simulink model "PS10_template2023"  (R2022b)
settings: Solver=ode45  StartTime=0.0  StopTime=10  FixedStep=.002  RelTol=1e-3  EnableMultiTasking=on
settings Model: ExtModeTrigDuration=10000  Creator=smascaro  LastModifiedBy=willg
settings SolverCC: AlgebraicLoopSolver=TrustRegion  PositivePriorityOrder=on
settings DataIOCC: SaveFormat=Array  SignalLoggingSaveFormat=ModelDataLogs  SaveOutput=off  SaveTime=off  ReturnWorkspaceOutputs=off
settings OptimizationCC: ExpressionDepthLimit=2147483647  InitFltsAndDblsToZero=on  LifeSpan=inf
settings DebuggingCC: SaveWithParameterizedLinksMsg=none  UnderspecifiedInitializationDetection=Classic  MergeDetectMultiDrivingBlocksExec=none  SignalResolutionControl=TryResolveAllWithWarning  SolverPrmCheckMsg=warning  MultiTaskDSMMsg=warning  MultiTaskCondExecSysMsg=none  FcnCallInpInsideContextMsg=warning  UnconnectedInputMsg=warning  UnconnectedOutputMsg=warning  UnconnectedLineMsg=warning  AllowSymbolicDim=off  StateNameClashWarn=warning  SFUnexpectedBacktrackingDiag=warning  SFNoUnconditionalDefaultTransitionDiag=warning  SFExecutionAtInitializationDiag=none  SFMachineParentedDataDiag=warning  ArithmeticOperatorsInVariantConditions=warning
settings HardwareCC: ProdBitPerPointer=32  ProdBitPerSizeT=32  ProdBitPerPtrDiffT=32  ProdLargestAtomicFloat=None  ProdIntDivRoundTo=Undefined  ProdEndianess=Unspecified  ProdWordSize=32  ProdHWDeviceType=32-bit Generic  TargetBitPerPointer=64  TargetBitPerSizeT=64  TargetBitPerPtrDiffT=64  TargetLongLongMode=on  TargetIntDivRoundTo=Zero  TargetEndianess=LittleEndian  TargetWordSize=64  TargetHWDeviceType=MATLAB Host
settings ModelReferenceCC: EnableRefExpFcnMdlSchedulingChecks=on  PropagateSignalLabelsOutOfModel=off
settings SFSimCC: SimUseLocalCustomCode=off  SimParseCustomCode=off  CustomCodeUndefinedFunction=UseInterfaceOnly
settings RTWCC: Description=QUARC Win32 Target  SystemTargetFile=quarc_windows.tlc  TemplateMakefile=quarc_default_tmf  RTWUseLocalCustomCode=off  DLArmComputeVersion=19.05
settings CodeAppCC: StateflowObjectComments=on
settings STFCustomTargetCC: TargetPreCompLibLocation=C:\PROGRA~3\QUARC\lib\2018a\windows\release  CPPClassGenCompliant=on  GRTInterface=on  SystemTargetFile=quarc_windows.tlc
settings GRTTargetCC: TargetPreCompLibLocation=C:\PROGRA~3\QUARC\lib\2018a\windows\release  TargetLangStandard=C89/C90 (ANSI)  ParMdlRefBuildCompliant=off  CompOptLevelCompliant=off  ConcurrentExecutionCompliant=off  CombineOutputUpdateFcns=off  MatFileLogging=off  GRTInterface=on  UseToolchainInfoCompliant=off  ExtMode=on  ExtModeMexFile=quarc_comm
settings ConfigComp: CovMetricSettings=dw  CovSaveCumulativeToWorkspaceVar=on  CovSaveSingleToWorkspaceVar=on  CovExternalEMLEnable=off

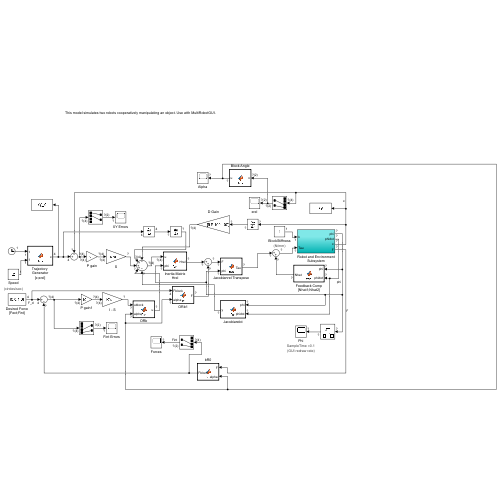
[thumbnail: Simulink's stored preview of the top-level diagram]
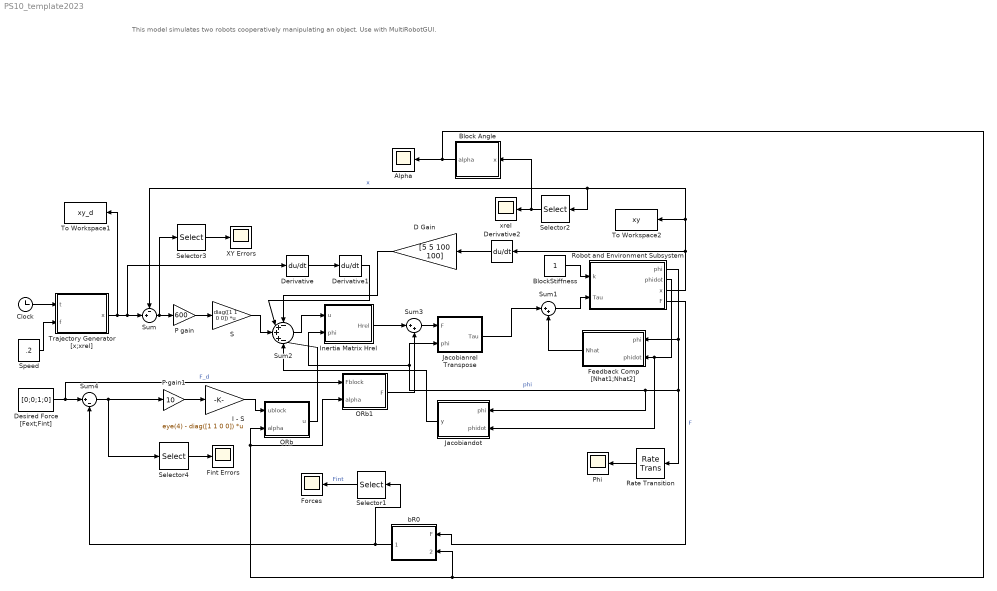
== system PS10_template2023 ==
  note: This model simulates two robots cooperatively manipulating an object. Use with MultiRobotGUI.
  Alpha : Scope
  Block Angle : MATLAB Function  TreatAsAtomicUnit=on
  BlockStiffness : Constant
      settings: AttributesFormatString=(N/mm)
  Clock : Clock
  D Gain : Gain  Gain=[5 5 100 100]
  Derivative : Derivative
  Derivative1 : Derivative
  Derivative2 : Derivative
  Desired Force [Fext;Fint] : Constant  Value=[0;0;1;0]
  Feedback Comp [Nhat1;Nhat2] : MATLAB Function  TreatAsAtomicUnit=on
  Fint Errors : Scope
  Forces : Scope
  I - S : Gain  Gain=eye(4) - diag([1 1 0 0])  Multiplication=Matrix(K*u)
  Inertia Matrix Hrel : MATLAB Function  TreatAsAtomicUnit=on
  Jacobiandot : MATLAB Function  TreatAsAtomicUnit=on
  Jacobianrel Transpose : MATLAB Function  TreatAsAtomicUnit=on
  ORb : MATLAB Function  TreatAsAtomicUnit=on
  ORb1 : MATLAB Function  TreatAsAtomicUnit=on
  P gain : Gain  Gain=600
  P gain1 : Gain  Gain=10
  Phi : Scope
      settings: AttributesFormatString=|
      | SampleTime =%<SampleTime>
      | (GUI redraw rate)
  Rate Transition : RateTransition  OutPortSampleTimeOpt=Inherit  OutPortSampleTimeMultiple=10  OutPortSampleTime=0.05
  Robot and Environment Subsystem : Subsystem
  S : Gain  Gain=diag([1 1 0 0])  Multiplication=Matrix(K*u)
  Selector1 : Selector  InputPortWidth=4  IndexOptions=Index vector (dialog)  Indices=[3 4]  OutputSizes=1
  Selector2 : Selector  InputPortWidth=4  IndexOptions=Index vector (dialog)  Indices=[3 4]  OutputSizes=1
  Selector3 : Selector  InputPortWidth=4  IndexOptions=Index vector (dialog)  Indices=[1 2]  OutputSizes=1
  Selector4 : Selector  InputPortWidth=4  IndexOptions=Index vector (dialog)  Indices=[3 4]  OutputSizes=1
  Speed : Constant  Value=.2
      settings: AttributesFormatString=(circles/sec)
  Sum : Sum  Inputs=-+|
  Sum1 : Sum  Inputs=|++
  Sum2 : Sum  Inputs=-+++-
  Sum3 : Sum  Inputs=|++
  Sum4 : Sum  Inputs=|+-
  To Workspace1 : ToWorkspace  VariableName=xy_d  SampleTime=-1
  To Workspace2 : ToWorkspace  VariableName=xy  SampleTime=-1
  Trajectory Generator [x;xrel] : MATLAB Function  TreatAsAtomicUnit=on
  XY Errors : Scope
  bR0 : MATLAB Function  TreatAsAtomicUnit=on
  xrel : Scope
  wires:
  Robot and Environment Subsystem/1(phi) -> Feedback Comp [Nhat1;Nhat2]/1(phi), Rate Transition/1, Jacobiandot/1(phi), Inertia Matrix Hrel/2(phi), Jacobianrel Transpose/2(phi)  "phi"
  Trajectory Generator [x;xrel]/1(x) -> To Workspace1/1, Derivative/1, Sum/2
  Robot and Environment Subsystem/3(x) -> Derivative2/1, To Workspace2/1, Sum/1, Selector2/1  "x"
  Clock/1 -> Trajectory Generator [x;xrel]/1(t)
  Speed/1 -> Trajectory Generator [x;xrel]/2(f)
  Rate Transition/1 -> Phi/1
  Robot and Environment Subsystem/4(F) -> bR0/1(F)  "F"
  Robot and Environment Subsystem/2(phidot) -> Jacobiandot/2(phidot), Feedback Comp [Nhat1;Nhat2]/2(phidot)
  Sum1/1 -> Robot and Environment Subsystem/2(Tau)
  BlockStiffness/1 -> Robot and Environment Subsystem/1(k)
  Desired Force [Fext;Fint]/1 -> ORb1/1(Fblock), Sum4/1  "F_d"
  Selector1/1 -> Forces/1  "Fint"
  Feedback Comp [Nhat1;Nhat2]/1(Nhat) -> Sum1/2
  Selector2/1 -> Block Angle/1(x), xrel/1
  Jacobianrel Transpose/1(Tau) -> Sum1/1
  Sum/1 -> Selector3/1, P gain/1
  Selector3/1 -> XY Errors/1
  Selector4/1 -> Fint Errors/1
  Sum4/1 -> P gain1/1, Selector4/1
  Derivative/1 -> Derivative1/1
  Derivative2/1 -> D Gain/1
  Sum3/1 -> Jacobianrel Transpose/1(F)
  Inertia Matrix Hrel/1(Hrel) -> Sum3/1
  Sum2/1 -> Inertia Matrix Hrel/1(u)
  D Gain/1 -> Sum2/1
  Derivative1/1 -> Sum2/2
  P gain/1 -> S/1
  P gain1/1 -> I - S/1
  S/1 -> Sum2/3
  Block Angle/1(alpha) -> ORb1/2(alpha), ORb/2(alpha), bR0/2(alpha), Alpha/1
  I - S/1 -> ORb/1(ublock)
  ORb/1(u) -> Sum2/4
  ORb1/1(F) -> Sum3/2
  Jacobiandot/1(y) -> Sum2/5
  bR0/1(Fblock) -> Selector1/1, Sum4/2

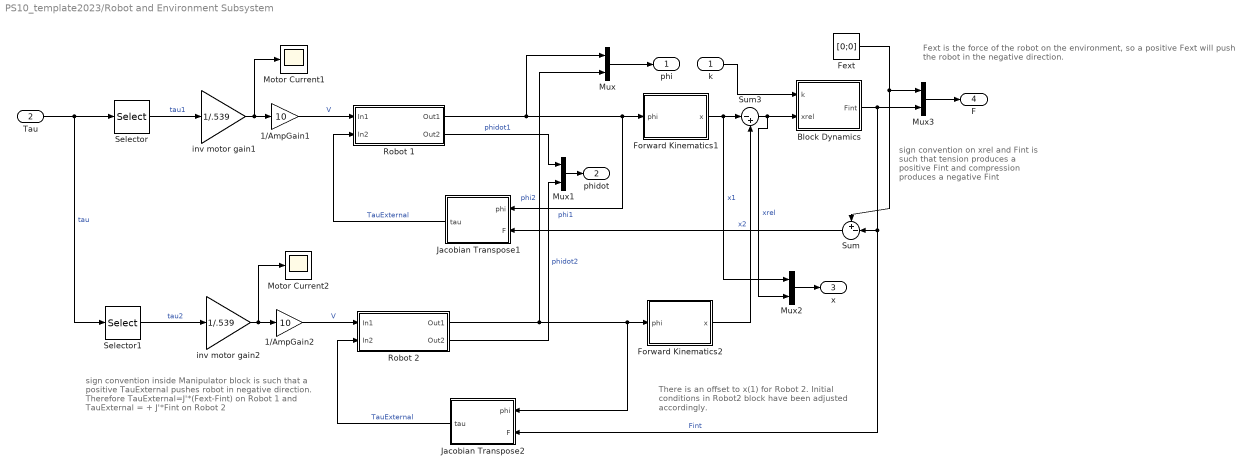
== system PS10_template2023/Robot and Environment Subsystem ==
  note: sign convention on xrel and Fint
      | is such that tension produces a positive Fint and compression produces a negative Fint
  note: There is an offset to x(1) for Robot 2. Initial
      | conditions in Robot2 block have been adjusted
      | accordingly.
  note: sign convention inside Manipulator block is such
      | that a positive TauExternal pushes robot in negative
      | direction. Therefore TauExternal=J'*(Fext-Fint) on Robot 1
      | and TauExternal = + J'*Fint on Robot 2
  note: Fext is the force of the robot on the environment, so a positive Fext will push the robot in the negative direction.
  k : Inport
  Tau : Inport  Port=2
  1/AmpGain1 : Gain  Gain=10
  1/AmpGain2 : Gain  Gain=10
  Block Dynamics : MATLAB Function  TreatAsAtomicUnit=on
  Fext : Constant  Value=[0;0]
  Forward Kinematics1 : MATLAB Function  TreatAsAtomicUnit=on
  Forward Kinematics2 : MATLAB Function  TreatAsAtomicUnit=on
  Jacobian Transpose1 : MATLAB Function  TreatAsAtomicUnit=on
  Jacobian Transpose2 : MATLAB Function  TreatAsAtomicUnit=on
  Motor Current1 : Scope
  Motor Current2 : Scope
  Mux{,1..3} (4 alike) : Mux  Inputs=2
  Robot 1 : Subsystem
      mask Display: disp('Manipulator')
  Robot 2 : Subsystem
      mask Display: disp('Manipulator')
  Selector : Selector  InputPortWidth=4  IndexOptions=Index vector (dialog)  Indices=[1 2]  OutputSizes=1
  Selector1 : Selector  InputPortWidth=4  IndexOptions=Index vector (dialog)  Indices=[3 4]  OutputSizes=1
  Sum : Sum  Inputs=+-|
  Sum3 : Sum  Inputs=|-+
  inv motor gain1 : Gain  Gain=1/.539
  inv motor gain2 : Gain  Gain=1/.539
  phi : Outport  VectorParamsAs1DForOutWhenUnconnected=off
  phidot : Outport  Port=2  VectorParamsAs1DForOutWhenUnconnected=off
  x : Outport  Port=3  VectorParamsAs1DForOutWhenUnconnected=off
  F : Outport  Port=4  VectorParamsAs1DForOutWhenUnconnected=off
  wires:
  Robot 1/1(Out1) -> Jacobian Transpose1/1(phi), Forward Kinematics1/1(phi), Mux/1  "phi1"
  Forward Kinematics1/1(x) -> Mux2/1, Sum3/1  "x1"
  inv motor gain1/1 -> 1/AmpGain1/1, Motor Current1/1
  1/AmpGain1/1 -> Robot 1/1(In1)  "V"
  k/1 -> Block Dynamics/1(k)
  Jacobian Transpose1/1(tau) -> Robot 1/2(In2)  "TauExternal"
  Robot 2/1(Out1) -> Jacobian Transpose2/1(phi), Forward Kinematics2/1(phi), Mux/2  "phi2"
  Forward Kinematics2/1(x) -> Sum3/2  "x2"
  inv motor gain2/1 -> 1/AmpGain2/1, Motor Current2/1
  1/AmpGain2/1 -> Robot 2/1(In1)  "V"
  Robot 2/2(Out2) -> Mux1/2  "phidot2"
  Selector1/1 -> inv motor gain2/1  "tau2"
  Jacobian Transpose2/1(tau) -> Robot 2/2(In2)  "TauExternal"
  Selector/1 -> inv motor gain1/1  "tau1"
  Tau/1 -> Selector/1, Selector1/1  "tau"
  Mux/1 -> phi/1
  Mux1/1 -> phidot/1
  Robot 1/2(Out2) -> Mux1/1  "phidot1"
  Mux3/1 -> F/1
  Fext/1 -> Mux3/1, Sum/1
  Mux2/1 -> x/1
  Sum3/1 -> Block Dynamics/2(xrel), Mux2/2  "xrel"
  Sum/1 -> Jacobian Transpose1/2(F)
  Block Dynamics/1(Fint) -> Jacobian Transpose2/2(F), Sum/2, Mux3/2  "Fint"

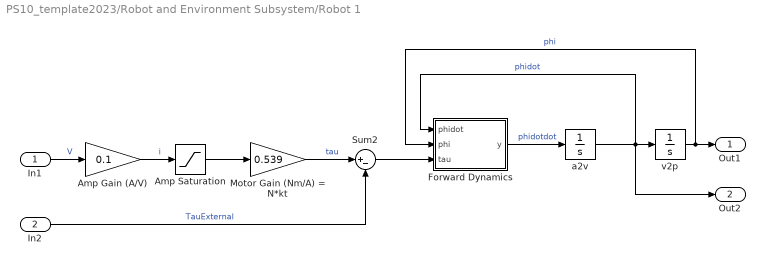
== system PS10_template2023/Robot and Environment Subsystem/Robot 1 ==
  In1 : Inport
  In2 : Inport  Port=2
  Amp Saturation : Saturate  UpperLimit=1  LowerLimit=-1  ZeroCross=off
  Amp Gain (A/V) : Gain  Gain=0.1
  Forward Dynamics : MATLAB Function  TreatAsAtomicUnit=on
  Motor Gain (Nm/A) = N*kt : Gain  Gain=0.539
  Sum2 : Sum  Inputs=|+-
  a2v : Integrator
  v2p : Integrator  InitialCondition=[1.1934;-0.2661]
  Out1 : Outport  VectorParamsAs1DForOutWhenUnconnected=off
  Out2 : Outport  Port=2  VectorParamsAs1DForOutWhenUnconnected=off
  wires:
  Forward Dynamics/1(y) -> a2v/1  "phidotdot"
  a2v/1 -> Out2/1, Forward Dynamics/1(phidot), v2p/1  "phidot"
  v2p/1 -> Out1/1, Forward Dynamics/2(phi)  "phi"
  In1/1 -> Amp Gain (A/V)/1  "V"
  Amp Saturation/1 -> Motor Gain (Nm/A) = N*kt/1
  Amp Gain (A/V)/1 -> Amp Saturation/1  "i"
  Sum2/1 -> Forward Dynamics/3(tau)
  Motor Gain (Nm/A) = N*kt/1 -> Sum2/1  "tau"
  In2/1 -> Sum2/2  "TauExternal"

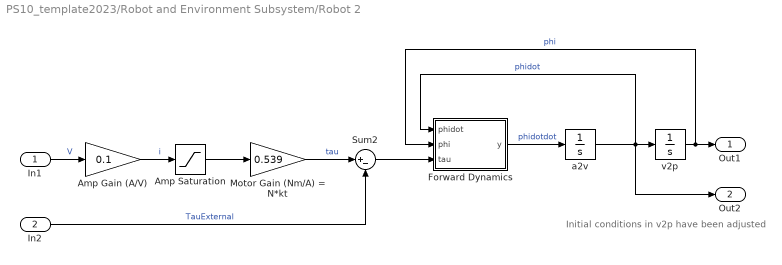
== system PS10_template2023/Robot and Environment Subsystem/Robot 2 ==
  note: Initial conditions in v2p have been adjusted
  In1 : Inport
  In2 : Inport  Port=2
  Amp Saturation : Saturate  UpperLimit=1  LowerLimit=-1  ZeroCross=off
  Amp Gain (A/V) : Gain  Gain=0.1
  Forward Dynamics : MATLAB Function  TreatAsAtomicUnit=on
  Motor Gain (Nm/A) = N*kt : Gain  Gain=0.539
  Sum2 : Sum  Inputs=|+-
  a2v : Integrator
  v2p : Integrator  InitialCondition=[pi-2.2961;pi+0.0818]
  Out1 : Outport  VectorParamsAs1DForOutWhenUnconnected=off
  Out2 : Outport  Port=2  VectorParamsAs1DForOutWhenUnconnected=off
  wires:
  Forward Dynamics/1(y) -> a2v/1  "phidotdot"
  a2v/1 -> Out2/1, Forward Dynamics/1(phidot), v2p/1  "phidot"
  v2p/1 -> Out1/1, Forward Dynamics/2(phi)  "phi"
  In1/1 -> Amp Gain (A/V)/1  "V"
  Amp Saturation/1 -> Motor Gain (Nm/A) = N*kt/1
  Amp Gain (A/V)/1 -> Amp Saturation/1  "i"
  Sum2/1 -> Forward Dynamics/3(tau)
  Motor Gain (Nm/A) = N*kt/1 -> Sum2/1  "tau"
  In2/1 -> Sum2/2  "TauExternal"

== matlab function PS10_template2023/Robot and Environment Subsystem/Jacobian Transpose1 ==
  settings: fimath=|
      | fimath(...
      | 'RoundMode', 'floor',...
      | 'OverflowMode', 'wrap',...
      | 'ProductMode', 'KeepLSB', 'ProductWordLength', 32,...
      | 'SumMode', 'KeepLSB', 'SumWordLength', 32,...
      | 'CastBeforeSum', false)
  data: tau output; phi input; F input
function tau = fcn(phi, F)
% This block supports an embeddable subset of the MATLAB language.
% See the help menu for details. 
a1=0.15;
a2=0.15;

J11 = -a1*sin(phi(1));
J12 = -a2*sin(phi(2));
J21 = a1*cos(phi(1));
J22 = a2*cos(phi(2));

J = [J11 J12; J21 J22];

tau = J'*F;

== matlab function PS10_template2023/ORb ==
  settings: fimath=|
      | fimath(...
      | 'RoundMode', 'floor',...
      | 'OverflowMode', 'wrap',...
      | 'ProductMode', 'KeepLSB', 'ProductWordLength', 32,...
      | 'SumMode', 'KeepLSB', 'SumWordLength', 32,...
      | 'CastBeforeSum', false)
  data: ublock input; u output; alpha input
function u = fcn(ublock, alpha)
% This block supports an embeddable subset of the MATLAB language.
% See the help menu for details. 
Rz = [cos(alpha), -sin(alpha); sin(alpha), cos(alpha)];

ubot = Rz*ublock(3:4);

u = [0 0 ubot(1) ubot(2)]';

== matlab function PS10_template2023/Block Angle ==
  settings: fimath=|
      | fimath(...
      | 'RoundMode', 'floor',...
      | 'OverflowMode', 'wrap',...
      | 'ProductMode', 'KeepLSB', 'ProductWordLength', 32,...
      | 'SumMode', 'KeepLSB', 'SumWordLength', 32,...
      | 'CastBeforeSum', false)
  data: alpha output; x input
function alpha = fcn(x)
% This block supports an embeddable subset of the MATLAB language.
% See the help menu for details. 


alpha = atan2(x(2), x(1));

== matlab function PS10_template2023/bR0 ==
  settings: fimath=|
      | fimath(...
      | 'RoundMode', 'floor',...
      | 'OverflowMode', 'wrap',...
      | 'ProductMode', 'KeepLSB', 'ProductWordLength', 32,...
      | 'SumMode', 'KeepLSB', 'SumWordLength', 32,...
      | 'CastBeforeSum', false)
  data: F input; Fblock output; alpha input
function Fblock = fcn(F, alpha)
% This block supports an embeddable subset of the MATLAB language.
% See the help menu for details. 
Rz = [cos(alpha), -sin(alpha); sin(alpha), cos(alpha)];
Fb = Rz'*F(3:4);


Fblock = [0 0 Fb(1) Fb(2)]';

== matlab function PS10_template2023/ORb1 ==
  settings: fimath=|
      | fimath(...
      | 'RoundMode', 'floor',...
      | 'OverflowMode', 'wrap',...
      | 'ProductMode', 'KeepLSB', 'ProductWordLength', 32,...
      | 'SumMode', 'KeepLSB', 'SumWordLength', 32,...
      | 'CastBeforeSum', false)
  data: Fblock input; F output; alpha input
function F = fcn(Fblock, alpha)
% This block supports an embeddable subset of the MATLAB language.
% See the help menu for details. 
Rz = [cos(alpha), -sin(alpha); sin(alpha), cos(alpha)];

Fint = Fblock(3:4);
Fbot = Rz*Fint;
F = [0 0 Fbot(1) Fbot(2)]';

== matlab function PS10_template2023/Robot and Environment Subsystem/Robot 1/Forward Dynamics ==
  settings: fimath=|
      | fimath(...
      | 'RoundMode', 'floor',...
      | 'OverflowMode', 'wrap',...
      | 'ProductMode', 'KeepLSB', 'ProductWordLength', 32,...
      | 'SumMode', 'KeepLSB', 'SumWordLength', 32,...
      | 'CastBeforeSum', false)
  data: phidot input double size=2; phi input double size=2; y output double size=2; tau input size=2
function y = fcn(phidot,phi,tau)
% This block supports an embeddable subset of the MATLAB language.
% See the help menu for details. 

a1 = 0.15;  % link 1 length
a2 = 0.15;  % link 2 length
m1 = 0.092;  % link 1 mass  
m2 = 0.077; % link 2 mas
r01 = 0.062; % link 1 center of mass
r12 = 0.036; % link 2 COM
I1 = 0.64e-3;  % link 1 inertia
I2 = 0.30e-3;  % link 2 inertia
Jm1 = 0.65e-6; % motor inertias
Jm2 = 0.65e-6;
b1 = 3.1e-6; % viscous damping constants
b2 = 3.1e-6;
c1 = 0.0001; % coulomb friction constants
c2 = 0.0001;
g = 9.8; % gravitational constant
N1 = 70; % gear ratios
N2 = 70;

H11 = N1^2*Jm1 + I1 + m2*a1^2;
H12 = a1*r12*m2*cos(phi(2)-phi(1));
H21 = H12;
H22 = N2^2*Jm2 + I2;
h = a1*r12*m2*sin(phi(2)-phi(1));
G1 = (r01*m1+a1*m2)*g*cos(phi(1));
G2 = r12*m2*g*cos(phi(2));
F1 = N1^2*b1*phidot(1) + N1*c1*sign(phidot(1));
F2 = N2^2*b2*phidot(2) + N2*c2*sign(phidot(2));

H = [H11 H12; H21 H22]; % inertia matrix
V = [0 -h ;h 0]*[phidot(1)^2;phidot(2)^2]; % centripetal torques
G = [G1;G2]; % gravity torques
F = [F1;F2]; % frictional torques

y = inv(H)*(tau - V - G - F); % y=phidotdot

== matlab function PS10_template2023/Inertia Matrix Hrel ==
  settings: fimath=|
      | fimath(...
      | 'RoundMode', 'floor',...
      | 'OverflowMode', 'wrap',...
      | 'ProductMode', 'KeepLSB', 'ProductWordLength', 32,...
      | 'SumMode', 'KeepLSB', 'SumWordLength', 32,...
      | 'CastBeforeSum', false)
  data: u input; phi input; Hrel output
function Hrel = fcn(u,phi)
% This block supports an embeddable subset of the MATLAB language.
% See the help menu for details. 


a1 = 0.15;  % link 1 length
a2 = 0.15;  % link 2 length
m1 = 0.092;  % link 1 mass  
m2 = 0.077; % link 2 mas
r01 = 0.062; % link 1 center of mass
r12 = 0.036; % link 2 COM
I1 = 0.64e-3;  % link 1 inertia
I2 = 0.30e-3;  % link 2 inertia
Jm1 = 0.65e-6; % motor inertias
Jm2 = 0.65e-6;

g = 9.8; % gravitational constant
N1 = 70; % gear ratios
N2 = 70;

H11 = N1^2*Jm1 + I1 + m2*a1^2;
H12 = a1*r12*m2*cos(phi(2)-phi(1));
H21 = H12;
H22 = N2^2*Jm2 + I2;

J11 = -a1*sin(phi(1));
J12 = -a2*sin(phi(2));
J21 = a1*cos(phi(1));
J22 = a2*cos(phi(2));

J_1 = [J11 J12; J21 J22];  %Jacobian 1

J11 = -a1*sin(phi(3));
J12 = -a2*sin(phi(4));
J21 = a1*cos(phi(3));
J22 = a2*cos(phi(4));

J_2 = [J11 J12; J21 J22]; % Jacobian 2

J = [J_1 zeros(2,2); -J_1 J_2]; %Relative Jacobian


H_1 = [H11 H12; H21 H22];  %Inertia Matrix in Joint Space robot 1

H11 = N1^2*Jm1 + I1 + m2*a1^2;
H12 = a1*r12*m2*cos(phi(4)-phi(3));
H21 = H12;
H22 = N2^2*Jm2 + I2;


H_2 = [H11 H12; H21 H22]; %Inertia Matrix in Joint Space robot 2

H = [H_1 zeros(2,2); H_2 zeros(2,2)];

Hx = inv(J')*H*inv(J);   %Inertia Matrix in Operational Space

Hrel = Hx*u;

== matlab function PS10_template2023/Feedback Comp [Nhat1;Nhat2] ==
  settings: fimath=|
      | fimath(...
      | 'RoundMode', 'floor',...
      | 'OverflowMode', 'wrap',...
      | 'ProductMode', 'KeepLSB', 'ProductWordLength', 32,...
      | 'SumMode', 'KeepLSB', 'SumWordLength', 32,...
      | 'CastBeforeSum', false)
  data: Nhat output; phi input; phidot input
function Nhat = fcn(phi, phidot)
% This block supports an embeddable subset of the MATLAB language.
% See the help menu for details. 


a1 = 0.15;  % link 1 length
a2 = 0.15;  % link 2 length
m1 = 0.092;  % link 1 mass  
m2 = 0.077; % link 2 mas
r01 = 0.062; % link 1 center of mass
r12 = 0.036; % link 2 COM
I1 = 0.64e-3;  % link 1 inertia
I2 = 0.30e-3;  % link 2 inertia
Jm1 = 0.65e-6; % motor inertias
Jm2 = 0.65e-6;
b1 = 3.1e-6; % viscous damping constants
b2 = 3.1e-6;
c1 = 0.0001; % coulomb friction constants
c2 = 0.0001;
g = 9.8; % gravitational constant
N1 = 70; % gear ratios
N2 = 70;

h = a1*r12*m2*sin(phi(2)-phi(1));
G1 = (r01*m1+a1*m2)*g*cos(phi(1));
G2 = r12*m2*g*cos(phi(2));
F1 = N1^2*b1*phidot(1) + N1*c1*sign(phidot(1));
F2 = N2^2*b2*phidot(2) + N2*c2*sign(phidot(2));

V = [0 -h ;h 0]*[phidot(1)^2;phidot(2)^2]; % centripetal torques
G = [G1;G2]; % gravity torques
F = [F1;F2]; % frictional torques

Nhat1 = (V + G + F);

h = a1*r12*m2*sin(phi(4)-phi(3));
G1 = (r01*m1+a1*m2)*g*cos(phi(3));
G2 = r12*m2*g*cos(phi(4));
F1 = N1^2*b1*phidot(3) + N1*c1*sign(phidot(3));
F2 = N2^2*b2*phidot(4) + N2*c2*sign(phidot(4));

V = [0 -h ;h 0]*[phidot(3)^2;phidot(4)^2]; % centripetal torques
G = [G1;G2]; % gravity torques
F = [F1;F2]; % frictional torques

Nhat2 = (V + G + F);

Nhat = [Nhat1;Nhat2];

== matlab function PS10_template2023/Robot and Environment Subsystem/Block Dynamics ==
  settings: fimath=|
      | fimath(...
      | 'RoundMode', 'floor',...
      | 'OverflowMode', 'wrap',...
      | 'ProductMode', 'KeepLSB', 'ProductWordLength', 32,...
      | 'SumMode', 'KeepLSB', 'SumWordLength', 32,...
      | 'CastBeforeSum', false)
  data: k input; xrel input; Fint output
function Fint = fcn(k,xrel)
% This block supports an embeddable subset of the MATLAB language.
% See the help menu for details. 

% kw = wall stiffness in N/mm, e.g. 1 N/mm

Fint = [0;0];

alpha = atan2(xrel(2),xrel(1));  % angle of block

d = sqrt(xrel(1)^2+xrel(2)^2);  % magnitude of xrel

F = k*1000*(d-0.1); % magnitude of force

Fint = [F*cos(alpha); F*sin(alpha)]; % form force vector in base frame

== matlab function PS10_template2023/Jacobianrel Transpose ==
  settings: fimath=|
      | fimath(...
      | 'RoundMode', 'floor',...
      | 'OverflowMode', 'wrap',...
      | 'ProductMode', 'KeepLSB', 'ProductWordLength', 32,...
      | 'SumMode', 'KeepLSB', 'SumWordLength', 32,...
      | 'CastBeforeSum', false)
  data: F input; Tau output; phi input
function Tau = fcn(F,phi)
% This block supports an embeddable subset of the MATLAB language.
% See the help menu for details. 
a1=0.15;
a2=0.15;

J11 = -a1*sin(phi(1));
J12 = -a2*sin(phi(2));
J21 = a1*cos(phi(1));
J22 = a2*cos(phi(2));

J1 = [J11 J12; J21 J22];

J11 = -a1*sin(phi(3));
J12 = -a2*sin(phi(4));
J21 = a1*cos(phi(3));
J22 = a2*cos(phi(4));



J2 = [J11 J12; J21 J22];


J_rel = [J1 zeros(2,2); -J1 J2];

Tau = J_rel'*F;

== matlab function PS10_template2023/Trajectory Generator [x;xrel] ==
  settings: fimath=|
      | fimath(...
      | 'RoundMode', 'floor',...
      | 'OverflowMode', 'wrap',...
      | 'ProductMode', 'KeepLSB', 'ProductWordLength', 32,...
      | 'SumMode', 'KeepLSB', 'SumWordLength', 32,...
      | 'CastBeforeSum', false)
  data: x output; t input; f input
function x = fcn(t,f)
% This block supports an embeddable subset of the MATLAB language.
% See the help menu for details. 
x = [0;0;0;0];

if t<0.5  % accelerate into circling trajectory
    x(1) = 0.075*cos(2*pi*f*t^2) + 0.125;
    x(2) = 0.075*sin(2*pi*f*t^2) + 0.1;
else  % constant speed circling of radius 0.075 about x=[0.125,0.1]
    x(1) = 0.075*cos(2*pi*f*(t-0.25)) + 0.125;
    x(2) = 0.075*sin(2*pi*f*(t-0.25)) + 0.1;
end
x(3) = 0.0; %desired relative x position of two robots
x(4) = 0.0; %desired relative y position of two robots

== matlab function PS10_template2023/Jacobiandot ==
  settings: fimath=|
      | fimath(...
      | 'RoundMode', 'floor',...
      | 'OverflowMode', 'wrap',...
      | 'ProductMode', 'KeepLSB', 'ProductWordLength', 32,...
      | 'SumMode', 'KeepLSB', 'SumWordLength', 32,...
      | 'CastBeforeSum', false)
  data: y output; phi input; phidot input
function y = fcn(phi, phidot)
% This block supports an embeddable subset of the MATLAB language.
% See the help menu for details. 
a1=0.15;
a2=0.15;

% J11 = -a1*sin(phi(1));
% J12 = -a2*sin(phi(2));
% J21 = a1*cos(phi(1));
% J22 = a2*cos(phi(2));

Jdot11 = -a1*cos(phi(1))*phidot(1);
Jdot12 = -a2*cos(phi(2))*phidot(2);
Jdot21 = -a1*sin(phi(1))*phidot(1);
Jdot22 = -a1*sin(phi(2))*phidot(2);

Jdot_1 = [Jdot11 Jdot12; Jdot21 Jdot22];

Jdot11 = -a1*cos(phi(3))*phidot(3);
Jdot12 = -a2*cos(phi(4))*phidot(4);
Jdot21 = -a1*sin(phi(3))*phidot(3);
Jdot22 = -a1*sin(phi(4))*phidot(4);

Jdot_2 = [Jdot11 Jdot12; Jdot21 Jdot22];


Jdot = [Jdot_1, zeros(2,2); -Jdot_1, Jdot_2];
y = Jdot*phidot;

== matlab function PS10_template2023/Robot and Environment Subsystem/Forward Kinematics1 ==
  settings: fimath=|
      | fimath(...
      | 'RoundMode', 'floor',...
      | 'OverflowMode', 'wrap',...
      | 'ProductMode', 'KeepLSB', 'ProductWordLength', 32,...
      | 'SumMode', 'KeepLSB', 'SumWordLength', 32,...
      | 'CastBeforeSum', false)
  data: x output; phi input
function x = fcn(phi)
% This block supports an embeddable subset of the MATLAB language.
% See the help menu for details. 

a1=0.15;
a2=0.15;
x = [0;0];
x(1) = a1*cos(phi(1))+a2*cos(phi(2));
x(2) = a1*sin(phi(1))+a2*sin(phi(2));

== matlab function PS10_template2023/Robot and Environment Subsystem/Forward Kinematics2 ==
  settings: fimath=|
      | fimath(...
      | 'RoundMode', 'floor',...
      | 'OverflowMode', 'wrap',...
      | 'ProductMode', 'KeepLSB', 'ProductWordLength', 32,...
      | 'SumMode', 'KeepLSB', 'SumWordLength', 32,...
      | 'CastBeforeSum', false)
  data: x output; phi input
function x = fcn(phi)
% This block supports an embeddable subset of the MATLAB language.
% See the help menu for details. 

a1=0.15;
a2=0.15;
x = [0;0];
x(1) = a1*cos(phi(1))+a2*cos(phi(2))+0.35;
x(2) = a1*sin(phi(1))+a2*sin(phi(2));

== matlab function PS10_template2023/Robot and Environment Subsystem/Jacobian Transpose2 ==
  settings: fimath=|
      | fimath(...
      | 'RoundMode', 'floor',...
      | 'OverflowMode', 'wrap',...
      | 'ProductMode', 'KeepLSB', 'ProductWordLength', 32,...
      | 'SumMode', 'KeepLSB', 'SumWordLength', 32,...
      | 'CastBeforeSum', false)
  data: tau output; phi input; F input
function tau = fcn(phi, F)
% This block supports an embeddable subset of the MATLAB language.
% See the help menu for details. 
a1=0.15;
a2=0.15;

J11 = -a1*sin(phi(1));
J12 = -a2*sin(phi(2));
J21 = a1*cos(phi(1));
J22 = a2*cos(phi(2));

J = [J11 J12; J21 J22];

tau = J'*F;

== matlab function PS10_template2023/Robot and Environment Subsystem/Robot 2/Forward Dynamics ==
  settings: fimath=|
      | fimath(...
      | 'RoundMode', 'floor',...
      | 'OverflowMode', 'wrap',...
      | 'ProductMode', 'KeepLSB', 'ProductWordLength', 32,...
      | 'SumMode', 'KeepLSB', 'SumWordLength', 32,...
      | 'CastBeforeSum', false)
  data: phidot input double size=2; phi input double size=2; y output double size=2; tau input size=2
function y = fcn(phidot,phi,tau)
% This block supports an embeddable subset of the MATLAB language.
% See the help menu for details. 

a1 = 0.15;  % link 1 length
a2 = 0.15;  % link 2 length
m1 = 0.092;  % link 1 mass  
m2 = 0.077; % link 2 mas
r01 = 0.062; % link 1 center of mass
r12 = 0.036; % link 2 COM
I1 = 0.64e-3;  % link 1 inertia
I2 = 0.30e-3;  % link 2 inertia
Jm1 = 0.65e-6; % motor inertias
Jm2 = 0.65e-6;
b1 = 3.1e-6; % viscous damping constants
b2 = 3.1e-6;
c1 = 0.0001; % coulomb friction constants
c2 = 0.0001;
g = 9.8; % gravitational constant
N1 = 70; % gear ratios
N2 = 70;

H11 = N1^2*Jm1 + I1 + m2*a1^2;
H12 = a1*r12*m2*cos(phi(2)-phi(1));
H21 = H12;
H22 = N2^2*Jm2 + I2;
h = a1*r12*m2*sin(phi(2)-phi(1));
G1 = (r01*m1+a1*m2)*g*cos(phi(1));
G2 = r12*m2*g*cos(phi(2));
F1 = N1^2*b1*phidot(1) + N1*c1*sign(phidot(1));
F2 = N2^2*b2*phidot(2) + N2*c2*sign(phidot(2));

H = [H11 H12; H21 H22]; % inertia matrix
V = [0 -h ;h 0]*[phidot(1)^2;phidot(2)^2]; % centripetal torques
G = [G1;G2]; % gravity torques
F = [F1;F2]; % frictional torques

y = inv(H)*(tau - V - G - F); % y=phidotdot
